simulink model "PID_AltSpeedController"  (Simulink 7.4)
settings: Solver=ode1  StartTime=0.0  StopTime=100  FixedStep=Ts  RelTol=1e-3
values from neighbouring files (symbols this model uses):
  P = modelo_quadrotor.solido.m*modelo_quadrotor.solido.g    [modelo.m]
  Vreferencia = 1    [modelo.m]
libraries: quadrotor_models x1, simulink x1
settings Model: Creator=g28115dq  LastModifiedBy=g28115dq

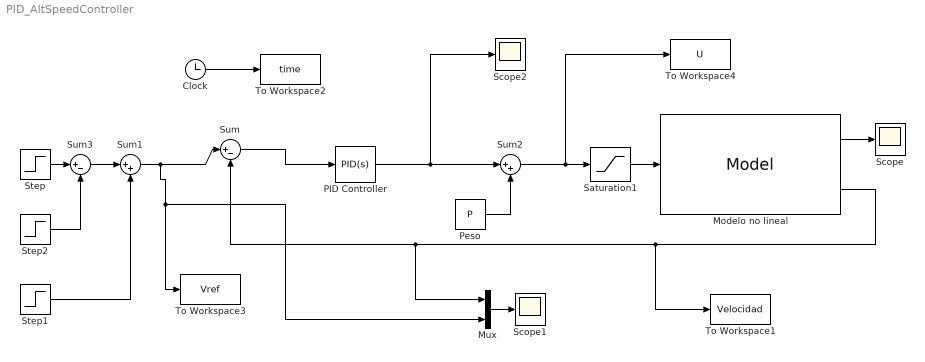
== system PID_AltSpeedController ==
  Clock : Clock
      settings: Decimation=10
  Modelo no lineal : quadrotor_models/Model  SystemSampleTime=-1
  Mux : Mux  Inputs=2
  PID Controller : simulink/Continuous/PID Controller  DialogController=pidpack.PIDConfig.pidDDGCreate  DialogControllerArgs=DataTag0  SystemSampleTime=-1  Controller=PID  TimeDomain=Continuous-time  SampleTime=1  IntegratorMethod=Forward Euler  FilterMethod=Forward Euler  Form=Parallel  P=3.2  I=2.56  D=0  N=100  InitialConditionSource=internal  InitialConditionForIntegrator=0  InitialConditionForFilter=0  ExternalReset=none  LimitOutput=on  UpperSaturationLimit=0.11*32  LowerSaturationLimit=-0.037*32  LinearizeAsGain=off  AntiWindupMode=clamping  Kb=1  TrackingMode=off  Kt=1  PParamMin=[]  PParamMax=[]  IParamMin=[]  IParamMax=[]  DParamMin=[]  DParamMax=[]  NParamMin=[]  NParamMax=[]  KbParamMin=[]  KbParamMax=[]  KtParamMin=[]  KtParamMax=[]  POutMin=[]  POutMax=[]  IOutMin=[]  IOutMax=[]  DOutMin=[]  DOutMax=[]  NOutMin=[]  NOutMax=[]  KbOutMin=[]  KbOutMax=[]  KtOutMin=[]  KtOutMax=[]  IntegratorOutMin=[]  IntegratorOutMax=[]  FilterOutMin=[]  FilterOutMax=[]  SumOutMin=[]  SumOutMax=[]  SumI1OutMin=[]  SumI1OutMax=[]  SumI2OutMin=[]  SumI2OutMax=[]  SumI3OutMin=[]  SumI3OutMax=[]  SumDOutMin=[]  SumDOutMax=[]  SaturationOutMin=[]  SaturationOutMax=[]  IntegratorContinuousStateAttributes=''  IntegratorStateMustResolveToSignalObject=off  IntegratorRTWStateStorageClass=Auto  FilterContinuousStateAttributes=''  FilterStateMustResolveToSignalObject=off  FilterRTWStateStorageClass=Auto
  Peso : Constant  Value=P  OutDataType=fixdt(1, 16)  OutScaling=2^0
  Saturation1 : Saturate  UpperLimit=32  LowerLimit=0  OutDataType=fixdt(1, 16)  OutScaling=2^0
  Scope : Scope
  Scope1 : Scope
      settings: TimeRange=30  YMin=-3.5  YMax=1.75
  Scope2 : Scope
      settings: TimeRange=30  SaveName=ScopeData2
  Step : Step  Time=50  After=Vreferencia  SampleTime=0
  Step1 : Step  Time=65  After=Vreferencia*0.5  SampleTime=0
  Step2 : Step  Time=80  After=Vreferencia*2.5  SampleTime=0
  Sum : Sum  Inputs=|+-  OutDataType=fixdt(1, 16)  OutScaling=2^0
  Sum1 : Sum  Inputs=|++  OutDataType=fixdt(1, 16)  OutScaling=2^0
  Sum2 : Sum  Inputs=|++  OutDataType=fixdt(1, 16)  OutScaling=2^0
  Sum3 : Sum  Inputs=|+-  OutDataType=fixdt(1, 16)  OutScaling=2^0
  To Workspace1 : ToWorkspace  VariableName=Velocidad  SampleTime=-1  SaveFormat=Array
  To Workspace2 : ToWorkspace  VariableName=time  SampleTime=-1  SaveFormat=Array
  To Workspace3 : ToWorkspace  VariableName=Vref  SampleTime=-1  SaveFormat=Array
  To Workspace4 : ToWorkspace  VariableName=U  SampleTime=-1  SaveFormat=Array
  wires:
  Sum1/1 -> Sum/1, To Workspace3/1, Mux/2
  Modelo no lineal/2 -> Mux/1, Sum/2, To Workspace1/1
  Modelo no lineal/1 -> Scope/1
  Mux/1 -> Scope1/1
  Clock/1 -> To Workspace2/1
  Step1/1 -> Sum1/2
  Peso/1 -> Sum2/2
  Sum3/1 -> Sum1/1
  Step/1 -> Sum3/1
  Step2/1 -> Sum3/2
  Sum/1 -> PID Controller/1
  Saturation1/1 -> Modelo no lineal/1
  Sum2/1 -> Saturation1/1, To Workspace4/1
  PID Controller/1 -> Scope2/1, Sum2/1
